simulink subsystem "rss_CrashFaltDia"  (R2023a)
settings: Solver=VariableStepAuto  StartTime=0.0  StopTime=10.0  RelTol=1e-3
undefined symbols (not defined in the file): ENM_TYPE_FALT, Gu16_ctCrashFaltConfCnt_C, Gu16_ctCrashFaltRcvyCnt_C
libraries: lib_debounce x1, lib_fault_definiteness x1
settings Model: Creator=xiaoqiang.yuan  LastModifiedBy=xiaoqiang.yuan

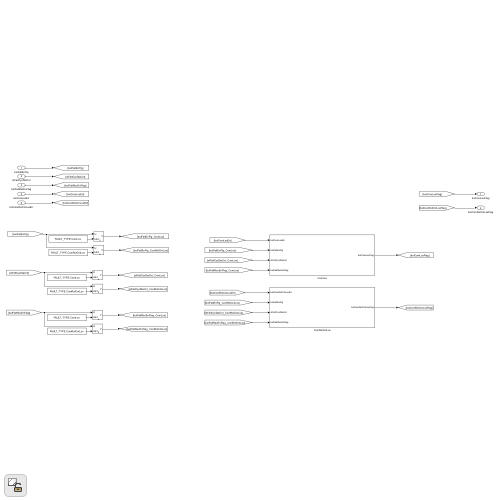
[thumbnail: Simulink's stored preview of the top-level diagram]
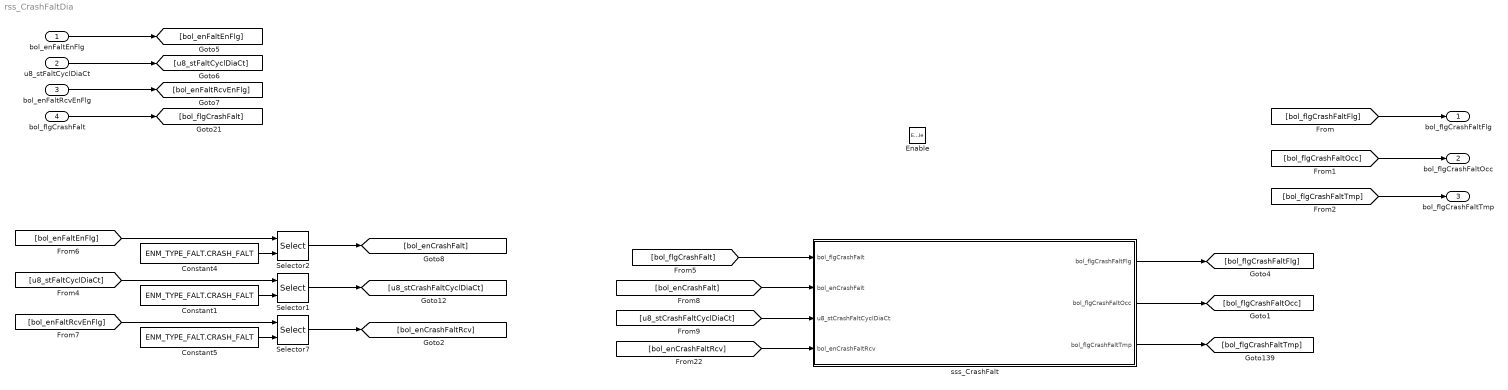
== system rss_CrashFaltDia ==
  bol_enFaltEnFlg : Inport  OutDataTypeStr=boolean
  u8_stFaltCyclDiaCt : Inport  Port=2  OutDataTypeStr=uint8
  bol_enFaltRcvEnFlg : Inport  Port=3  OutDataTypeStr=boolean
  bol_flgCrashFalt : Inport  Port=4  OutDataTypeStr=boolean
  Enable : EnablePort
  Constant1 : Constant  Value=ENM_TYPE_FALT.CRASH_FALT
  Constant4 : Constant  Value=ENM_TYPE_FALT.CRASH_FALT
  Constant5 : Constant  Value=ENM_TYPE_FALT.CRASH_FALT
  Selector1 : Selector  IndexMode=Zero-based  InputPortWidth=Cdbl_numFaltDiaNum  IndexOptions=Index vector (port)  Indices=[1 3]  OutputSizes=1
  Selector2 : Selector  IndexMode=Zero-based  InputPortWidth=Cdbl_numFaltDiaNum  IndexOptions=Index vector (port)  Indices=[1 3]  OutputSizes=1
  Selector7 : Selector  IndexMode=Zero-based  InputPortWidth=Cdbl_numFaltDiaNum  IndexOptions=Index vector (port)  Indices=[1 3]  OutputSizes=1
  sss_CrashFalt : Subsystem
  bol_flgCrashFaltFlg : Outport  OutDataTypeStr=boolean
  bol_flgCrashFaltOcc : Outport  Port=2  OutDataTypeStr=boolean
  bol_flgCrashFaltTmp : Outport  Port=3  OutDataTypeStr=boolean
  wires:
  [bol_flgCrashFaltFlg] -> bol_flgCrashFaltFlg/1
  [u8_stFaltCyclDiaCt] -> Selector1/1
  [bol_enFaltEnFlg] -> Selector2/1
  bol_enFaltEnFlg/1 -> [bol_enFaltEnFlg]
  bol_enFaltRcvEnFlg/1 -> [bol_enFaltRcvEnFlg]
  [bol_flgCrashFalt] -> sss_CrashFalt/1(bol_flgCrashFalt)
  Constant1/1 -> Selector1/2
  [u8_stCrashFaltCyclDiaCt] -> sss_CrashFalt/3(u8_stCrashFaltCyclDiaCt)
  [bol_enCrashFalt] -> sss_CrashFalt/2(bol_enCrashFalt)
  Constant4/1 -> Selector2/2
  Constant5/1 -> Selector7/2
  Selector1/1 -> [u8_stCrashFaltCyclDiaCt]
  bol_flgCrashFalt/1 -> [bol_flgCrashFalt]
  Selector7/1 -> [bol_enCrashFaltRcv]
  [bol_enFaltRcvEnFlg] -> Selector7/1
  Selector2/1 -> [bol_enCrashFalt]
  [bol_enCrashFaltRcv] -> sss_CrashFalt/4(bol_enCrashFaltRcv)
  u8_stFaltCyclDiaCt/1 -> [u8_stFaltCyclDiaCt]
  sss_CrashFalt/1(bol_flgCrashFaltFlg) -> [bol_flgCrashFaltFlg]
  sss_CrashFalt/2(bol_flgCrashFaltOcc) -> [bol_flgCrashFaltOcc]
  [bol_flgCrashFaltOcc] -> bol_flgCrashFaltOcc/1
  [bol_flgCrashFaltTmp] -> bol_flgCrashFaltTmp/1
  sss_CrashFalt/3(bol_flgCrashFaltTmp) -> [bol_flgCrashFaltTmp]

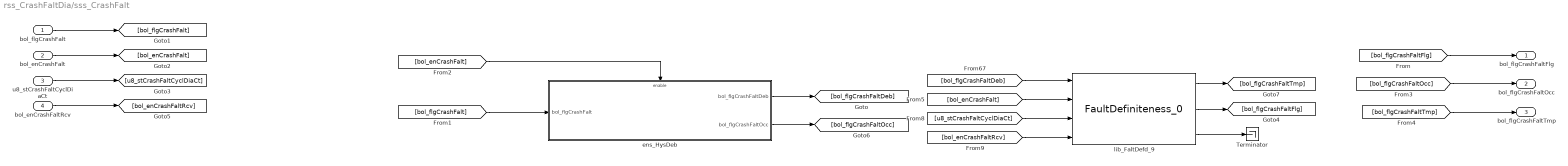
== system rss_CrashFaltDia/sss_CrashFalt ==
  bol_flgCrashFalt : Inport
  bol_enCrashFalt : Inport  Port=2
  u8_stCrashFaltCyclDiaCt : Inport  Port=3
  bol_enCrashFaltRcv : Inport  Port=4
  Terminator : Terminator
  ens_HysDeb : Subsystem
  lib_FaltDefd_9 : lib_fault_definiteness/FaultDefiniteness_0  lb_FaltWaitRecvCnt=Gu16_ctCrashFaltConfCnt_C
  bol_flgCrashFaltFlg : Outport
  bol_flgCrashFaltOcc : Outport  Port=2
  bol_flgCrashFaltTmp : Outport  Port=3
  wires:
  [bol_flgCrashFaltTmp] -> bol_flgCrashFaltTmp/1
  [bol_flgCrashFaltOcc] -> bol_flgCrashFaltOcc/1
  ens_HysDeb/2(bol_flgCrashFaltOcc) -> [bol_flgCrashFaltOcc]
  lib_FaltDefd_9/1 -> [bol_flgCrashFaltTmp]
  lib_FaltDefd_9/2 -> [bol_flgCrashFaltFlg]
  lib_FaltDefd_9/3 -> Terminator/1
  [bol_enCrashFalt] -> ens_HysDeb/Enable
  [bol_flgCrashFalt] -> ens_HysDeb/1(bol_flgCrashFalt)
  ens_HysDeb/1(bol_flgCrashFaltDeb) -> [bol_flgCrashFaltDeb]
  bol_enCrashFaltRcv/1 -> [bol_enCrashFaltRcv]
  u8_stCrashFaltCyclDiaCt/1 -> [u8_stCrashFaltCyclDiaCt]
  bol_enCrashFalt/1 -> [bol_enCrashFalt]
  [bol_flgCrashFaltFlg] -> bol_flgCrashFaltFlg/1
  bol_flgCrashFalt/1 -> [bol_flgCrashFalt]
  [bol_enCrashFaltRcv] -> lib_FaltDefd_9/4
  [u8_stCrashFaltCyclDiaCt] -> lib_FaltDefd_9/3
  [bol_enCrashFalt] -> lib_FaltDefd_9/2
  [bol_flgCrashFaltDeb] -> lib_FaltDefd_9/1

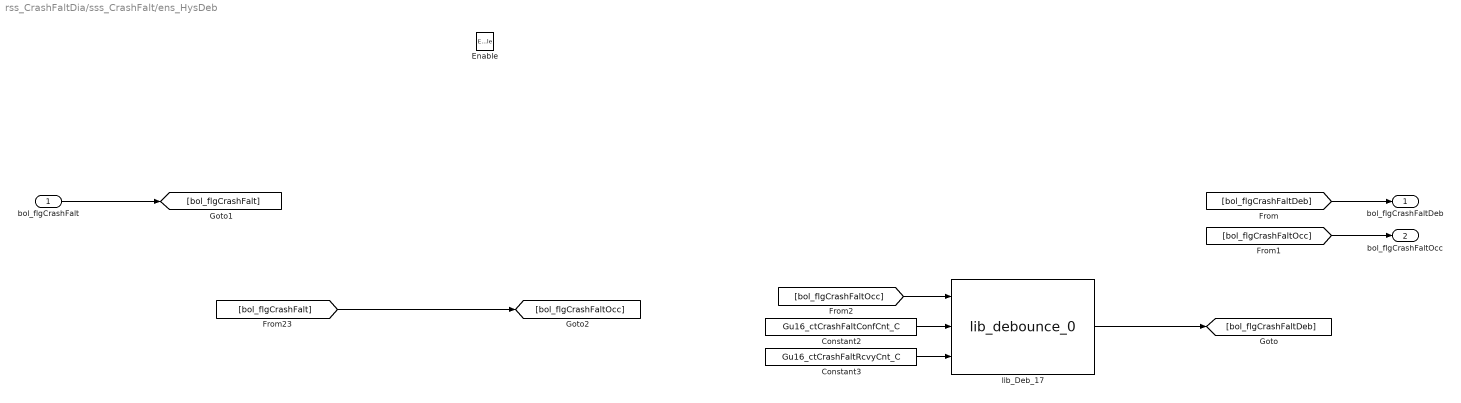
== system rss_CrashFaltDia/sss_CrashFalt/ens_HysDeb ==
  bol_flgCrashFalt : Inport
  Enable : EnablePort
  Constant2 : Constant  Value=Gu16_ctCrashFaltConfCnt_C
  Constant3 : Constant  Value=Gu16_ctCrashFaltRcvyCnt_C
  lib_Deb_17 : lib_debounce/lib_debounce_0
  bol_flgCrashFaltDeb : Outport
  bol_flgCrashFaltOcc : Outport  Port=2
  wires:
  [bol_flgCrashFaltOcc] -> lib_Deb_17/1
  [bol_flgCrashFalt] -> [bol_flgCrashFaltOcc]
  [bol_flgCrashFaltOcc] -> bol_flgCrashFaltOcc/1
  lib_Deb_17/1 -> [bol_flgCrashFaltDeb]
  bol_flgCrashFalt/1 -> [bol_flgCrashFalt]
  [bol_flgCrashFaltDeb] -> bol_flgCrashFaltDeb/1
  Constant3/1 -> lib_Deb_17/3
  Constant2/1 -> lib_Deb_17/2
